simulink model "DTW"  (R2017b)
settings: Solver=VariableStepAuto  StartTime=0.0  StopTime=45.0  RelTol=1e-3
libraries: hdlsllib x5
settings Model: Creator=V  LastModifiedBy=V

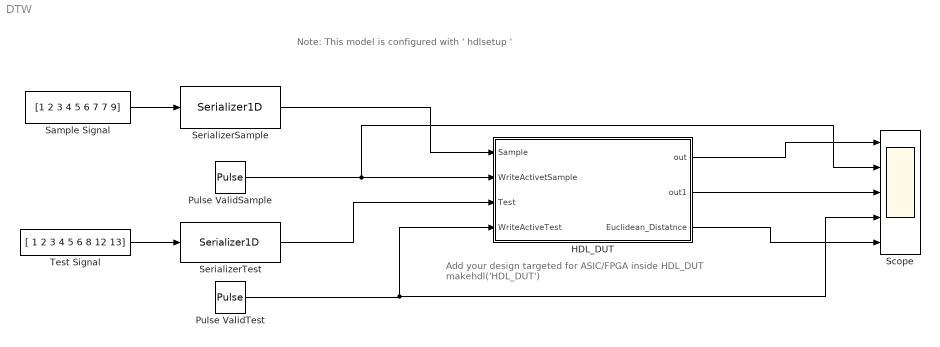
== system DTW ==
  note: Note: This model is configured with ' hdlsetup '
  note: Add your design targeted for ASIC/FPGA inside HDL_DUT
      | makehdl('HDL_DUT')
  HDL_DUT : Subsystem
  Pulse ValidSample : DiscretePulseGenerator
  Pulse ValidTest : DiscretePulseGenerator
  Sample Signal : Constant  Value=[1 2 3 4 5 6 7 7 9]  OutDataTypeStr=int16  SampleTime=1
  Scope : Scope  NumInputPorts=5
  "SerializerSample " : hdlsllib/HDL Operations/Serializer1D  Ratio=9  IdleCycles=0  validIn=off  startOut=off  validOut=off  inputDataDimensions=-1  inputSampleTime=-1  inputSignalType=auto
      settings: SourceProductName=HDL Coder  SourceProductBaseCode=HD
  "SerializerTest " : hdlsllib/HDL Operations/Serializer1D  Ratio=9  IdleCycles=0  validIn=off  startOut=off  validOut=off  inputDataDimensions=-1  inputSampleTime=-1  inputSignalType=auto
      settings: SourceProductName=HDL Coder  SourceProductBaseCode=HD
  Test Signal : Constant  Value=[ 1 2 3 4 5 6 8 12 13]  OutDataTypeStr=int16  SampleTime=1
  wires:
  Pulse ValidSample/1 -> Scope/2, HDL_DUT/2(WriteActivetSample)
  "SerializerSample "/1 -> HDL_DUT/1("Sample ")
  Sample Signal/1 -> "SerializerSample "/1
  Pulse ValidTest/1 -> Scope/4, HDL_DUT/4(WriteActiveTest)
  HDL_DUT/1(out) -> Scope/1
  "SerializerTest "/1 -> HDL_DUT/3(Test)
  HDL_DUT/2(out1) -> Scope/3
  Test Signal/1 -> "SerializerTest "/1
  HDL_DUT/3("Euclidean_Distatnce ") -> Scope/5

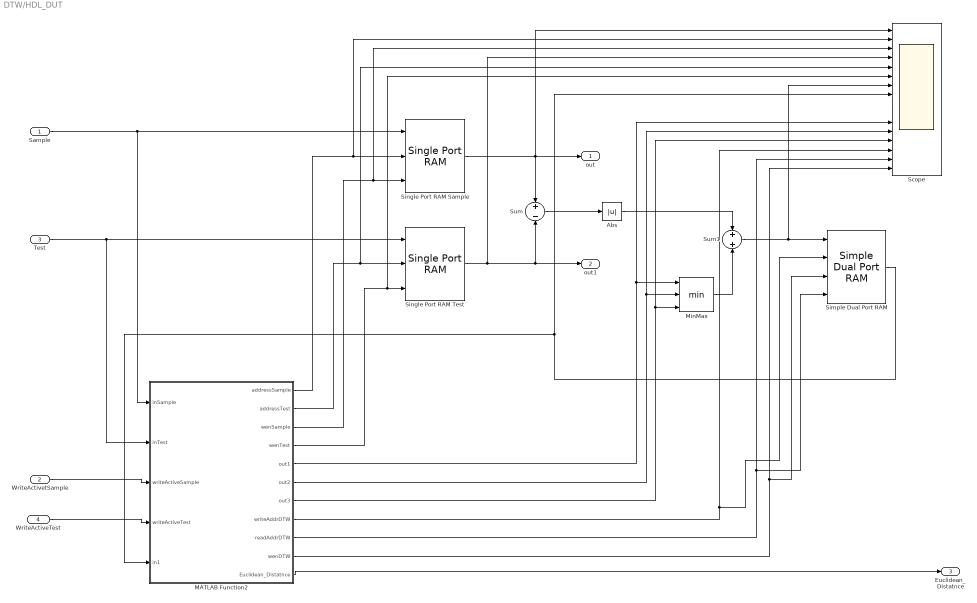
== system DTW/HDL_DUT ==
  "Sample " : Inport  Description=Sample
  WriteActivetSample : Inport  Port=2
  Test : Inport  Port=3
  WriteActiveTest : Inport  Port=4
  Abs : Abs  OutDataTypeStr=uint8
  MATLAB Function2 : MATLAB Function  TreatAsAtomicUnit=on
  MinMax : MinMax  Inputs=3  OutDataTypeStr=uint8
  Scope : Scope  NumInputPorts=16
  Simple Dual Port RAM : hdlsllib/HDL RAMs/Simple Dual Port RAM  ram_size=16
      settings: SourceProductName=HDL Coder  SourceProductBaseCode=HD
  Single Port RAM Sample : hdlsllib/HDL RAMs/Single Port RAM  ram_size=16  dout_type=New data
      settings: SourceProductName=HDL Coder  SourceProductBaseCode=HD
  "Single Port RAM Test " : hdlsllib/HDL RAMs/Single Port RAM  ram_size=16  dout_type=New data
      settings: SourceProductName=HDL Coder  SourceProductBaseCode=HD
  Sum : Sum  Inputs=+-  OutDataTypeStr=int8  SaturateOnIntegerOverflow=on
  Sum1 : Sum  SaturateOnIntegerOverflow=on
  out : Outport
  out1 : Outport  Port=2
  "Euclidean_Distatnce " : Outport  Port=3
  wires:
  MATLAB Function2/7(out3) -> Scope/13, MinMax/3
  Simple Dual Port RAM/1 -> Scope/8, MATLAB Function2/5(in1)
  "Single Port RAM Test "/1 -> Scope/4, out1/1, Sum/2
  WriteActivetSample/1 -> MATLAB Function2/3(writeActiveSample)
  MATLAB Function2/6(out2) -> Scope/12, MinMax/2
  MATLAB Function2/1(addressSample) -> Scope/2, Single Port RAM Sample/2
  MATLAB Function2/9(readAddrDTW) -> Scope/15, Simple Dual Port RAM/4
  Test/1 -> MATLAB Function2/2(inTest), "Single Port RAM Test "/1
  MATLAB Function2/5(out1) -> MinMax/1, Scope/11
  MinMax/1 -> Sum1/2
  MATLAB Function2/8(writeAddrDTW) -> Scope/14, Simple Dual Port RAM/2
  MATLAB Function2/10(wenDTW) -> Scope/16, Simple Dual Port RAM/3
  Sum/1 -> Abs/1
  Sum1/1 -> Scope/7, Simple Dual Port RAM/1
  MATLAB Function2/11(Euclidean_Distatnce) -> "Euclidean_Distatnce "/1
  MATLAB Function2/3(wenSample) -> Scope/3, Single Port RAM Sample/3
  MATLAB Function2/4(wenTest) -> Scope/6, "Single Port RAM Test "/3
  WriteActiveTest/1 -> MATLAB Function2/4(writeActiveTest)
  "Sample "/1 -> Single Port RAM Sample/1, MATLAB Function2/1(inSample)
  Abs/1 -> Sum1/1
  Single Port RAM Sample/1 -> Scope/1, out/1, Sum/1
  MATLAB Function2/2(addressTest) -> Scope/5, "Single Port RAM Test "/2

== matlab function DTW/HDL_DUT/MATLAB Function2 ==
  data: inSample input; inTest input; writeActiveSample input; writeActiveTest input; addressSample output uint16; addressTest output uint16; wenSample output; wenTest output; in1 input; out1 output; out2 output; out3 output; writeAddrDTW output; readAddrDTW output; wenDTW output; Euclidean_Distatnce output
function [addressSample, addressTest, wenSample , wenTest ,out1 , out2 , out3, writeAddrDTW, readAddrDTW, wenDTW, Euclidean_Distatnce]= fcn(inSample, inTest, writeActiveSample , writeActiveTest, in1)
 persistent addrSample;
 persistent addrTest; 
 persistent calcStart;    %% a flag, when receiving input signals completed, it will be = 1
 persistent wenTestPer;
 persistent wenSamplePer;
 persistent writeSampleFinish;
 persistent writeTestFinish;
 persistent flagNextRow;
 persistent validCalcPer; 
 persistent writeAddr; 
 persistent readAddr;
 persistent temp1;
 persistent temp2;
 persistent temp3;
 persistent wen;
 persistent Euclidean_DistatncePer;
 persistent startWrite;
 persistent startRead;
 persistent count;
 persistent validTemp;
 persistent validMin;
 persistent readNextPer;
 persistent numTest;
 persistent numSample;
 persistent numDTWMatrix; 
 persistent writeSampleHasRun;
 persistent writeTestHasRun;
 persistent validTest;
 persistent validSample;
 if isempty(numDTWMatrix)
      numDTWMatrix= ufi(0,16,0);
 end
 if isempty(validTest)
      validTest= ufi(0,1,0);
 end
 if isempty(validSample)
      validSample= ufi(0,1,0);
 end
 if isempty(writeSampleHasRun)
      writeSampleHasRun= ufi(0,1,0);
 end
  if isempty(writeTestHasRun)
      writeTestHasRun= ufi(0,1,0);
  end
  if isempty(writeSampleFinish)
      writeSampleFinish= ufi(0,1,0);
  end
  if isempty(writeTestFinish)
      writeTestFinish=ufi(0,1,0);
  end
  if isempty(wenTestPer)
      wenTestPer=ufi(0,1,0);
  end
  if isempty(wenSamplePer)
      wenSamplePer=ufi(0,1,0);
  end
  if isempty(calcStart)
      calcStart=ufi(0,1,0);
  end
  if isempty(addrSample)
      addrSample=ufi(0,16,0);
  end
  if isempty(addrTest)
      addrTest=ufi(0,16,0);
  end
  if isempty(flagNextRow)
      flagNextRow= ufi(0,1,0);
  end
  if isempty(validCalcPer)
      validCalcPer= ufi(0,1,0);
  end
  if isempty(writeAddr)        %% ----------  initializing persitents
      writeAddr= ufi(0,16,0);
  end
  if isempty(readAddr)
      readAddr= ufi(0,16,0);
  end
  if isempty(temp1)
      temp1= sfi(0,16,0);
  end
  if isempty(temp2)
      temp2= sfi(0,16,0);
  end
  if isempty(temp3)
      temp3= sfi(0,16,0);
  end
  if isempty(wen)
      wen= ufi(0,1,0);
  end
  if isempty(Euclidean_DistatncePer)
      Euclidean_DistatncePer= sfi(0,16,0);
  end
  if isempty(startWrite)
      startWrite= ufi(0,1,0);
  end
  if isempty(startRead)
      startRead= ufi(0,1,0);
  end
  if isempty(count)
      count= ufi(0,16,0);
  end
  if isempty(validTemp)
      validTemp= ufi(0,1,0);
  end
  if isempty(validMin)
      validMin= ufi(0,1,0);
  end
   if isempty(readNextPer)
      readNextPer= ufi(0,1,0);
   end
   if isempty(numSample)
      numSample= ufi(0,16,0);
   end
   if isempty(numTest)
      numTest= ufi(0,16,0);
   end
%----------------------------------------------------- Sample and Test block
 %%%---------------------------------------  Start Reading Test & sample
  %%%Matrix elements
  if(readNextPer)  %% inja  writeTestFinish && writeSampleFinish &&
      readNextPer = ufi(0,1,0);
      validCalcPer = ufi(1,1,0);
     if(addrTest < uint16(numTest+1))      
        addrTest = ufi(addrTest +1,16,0);  
     end
     if(addrTest == uint16(numTest+1))
        addrTest = ufi(1,16,0);   
        flagNextRow = ufi (1,1,0);
     end     
      
     if(flagNextRow && addrSample < uint16(numSample+1)) 
        addrSample = ufi(addrSample +1,16,0); 
        flagNextRow = ufi(0,1,0);
     end
     if(addrSample == uint16(numSample+1))
        addrSample = ufi(1,16,0);    
     end   
     
  end 

   %%------------------- writing Test and sample signals into Sample and Test Rams  
   %%--------------------  Sample:
  if(writeActiveSample && writeSampleFinish == 0)
      writeSampleHasRun = ufi(1,1,0);
    if(inSample > int16(2))                          % threshold for removing silence
        addrSample = ufi( addrSample + 1 , 16 , 0);
        wenSamplePer=ufi(1,1,0);
    else
        wenSamplePer=ufi(0,1,0);                 
    end    
  end
  
  if(writeSampleHasRun && writeActiveSample == 0)
     writeSampleHasRun=ufi(0,1,0);
     writeSampleFinish = ufi(1,1,0);
     wenSamplePer= ufi(0,1,0);
     numSample = ufi(addrSample ,16 ,0);
     addrSample = ufi(1 ,16 ,0);
     validSample = ufi(1,1,0);
  end
%%-------------------------------------------  Test:
  if(writeActiveTest && writeTestFinish == 0)
    writeTestHasRun = ufi(1,1,0); 
    if(inTest > int16(2))
        addrTest = ufi( addrTest +1 , 16 ,0); 
        wenTestPer = ufi(1,1,0);
    else
        wenTestPer = ufi(0,1,0);
    end   
  end
  
  if(writeTestHasRun && writeActiveTest == 0)
      writeTestHasRun=ufi(0,1,0);
      writeTestFinish=ufi(1,1,0);
      wenTestPer = ufi(0,1,0);
      numTest=ufi(addrTest,16,0);
      addrTest = ufi( 1,16,0); 
      validTest=ufi(1,1,0);
  end
 %%--------------------------------------- finish receiving Test and Sample 
  if(validTest && validSample)
      validTest=ufi(0,1,0);
      validSample=ufi(0,1,0);
      numDTWMatrix = ufi( (numTest*numSample),16,0);
      validCalcPer = ufi(1,1,0);  
  end
  
  if(writeTestFinish)
      wenTestPer = ufi(0,1,0);
  end
  if(writeSampleFinish)
      wenSamplePer= ufi(0,1,0);
  end 
 
  
% ------------------------------------------ Start Calculating DTW Ram
  if(validCalcPer)
    validCalcPer = ufi(0,1,0);
    startRead = ufi(1,1,0);
  end

  if(wen && writeAddr < uint16(numDTWMatrix) )      %%--------------------------  writing Block 
      readNextPer = ufi(1,1,0);
      wen = ufi(0,1,0);
      writeAddr = ufi(writeAddr+1 , 16 ,0);
  elseif(writeAddr == uint16(numDTWMatrix))
     readAddr = ufi(numDTWMatrix-1 ,16,0);
     wen = ufi(0,1,0);
     Euclidean_DistatncePer = sfi(in1,16,0);
  end
  
  if(validMin)
      validMin = ufi(0,1,0);
      wen = ufi(1,1,0); 
  end
  
    if(validTemp) 
       startRead = ufi(0,1,0);
       validTemp = ufi(0,1,0);
      if(addrSample == uint16(1))
          if(addrTest== uint16(1))
             temp1 = sfi(0,16,0);
             temp2 = sfi(100,16,0);
             temp3 = sfi(100,16,0);
             validMin = ufi(1,1,0);
          else
             temp1 = sfi(100,16,0);
             temp2 = sfi(100,16,0);
             validMin = ufi(1,1,0);
          end  
          
      else
          if(addrTest == uint8(1))
             temp1 = sfi(100,16,0);
             temp3 = sfi(100,16,0);
             validMin = ufi(1,1,0);
          else
             validMin = ufi(1,1,0);
          end       
      end  
   end 
  
    if(startRead && writeAddr < uint16(numDTWMatrix))    %% --------------- reading block
        if(count==uint16(0))
            count = ufi(count + 1 ,16 ,0);
            readAddr = ufi(writeAddr-1,16,0);
        elseif(count == uint16(1))
             temp3= sfi(in1,16,0);
             count = ufi(count + 1 ,16 ,0);
             readAddr = ufi(readAddr - numTest+1 , 16, 0);
        elseif(count == uint16(2))
            temp2= sfi(in1,16,0);
            count = ufi(count + 1 ,16 ,0);
            readAddr = ufi(readAddr - 1 , 16, 0);
        elseif(count == uint16(3))
            temp1= sfi(in1,16,0);
            count = ufi(0,16,0);
            validTemp = ufi(1,1,0);
        end    
    end     
  
 
 addressSample = uint16(addrSample);
 addressTest = uint16(addrTest);
 wenSample = logical(wenSamplePer);
 wenTest = logical(wenTestPer);
 out1 = int16(temp1);
 out2 = int16(temp2);
 out3 = int16(temp3);
 writeAddrDTW = uint16(writeAddr);
 readAddrDTW = uint16(readAddr);
 wenDTW = logical(wen);
 Euclidean_Distatnce = int16(Euclidean_DistatncePer); 
end
